simulink model "Quadrotor_model_2020_PID_R2025a"  (R2025a)
settings: Solver=FixedStepDiscrete  StartTime=0.0  StopTime=q2020_t_stop  FixedStep=pid_dt  RelTol=1e-3  EnableMultiTasking=on
InitFcn:
  | run('C:\00_Research_\Neuromorphic_Embodied_AI\02_Coaxial_TriRotor_Nengo\baseline_victor\PID_R2025a_models\params\victor_pid_params.m')
undefined symbols (not defined in the file): pid_dt, q2020_int0, q2020_param_vec, q2020_x0
settings Model: ExtModeTrigDuration=10000  Creator=gandhico  LastModifiedBy=gandhico
settings SolverCC: AlgebraicLoopSolver=TrustRegion  PositivePriorityOrder=on
settings DataIOCC: ReturnWorkspaceOutputs=off
settings DebuggingCC: UnconnectedInputMsg=warning  UnconnectedOutputMsg=warning  UnconnectedLineMsg=warning  ArithmeticOperatorsInVariantConditions=warning
settings ModelReferenceCC: EnableRefExpFcnMdlSchedulingChecks=on
settings SFSimCC: SimUseLocalCustomCode=off  CustomCodeUndefinedFunction=UseInterfaceOnly
settings RTWCC: SystemTargetFile=quarc_win64.tlc  TemplateMakefile=quarc_default_tmf  RTWUseLocalCustomCode=off  Toolchain=QUARC win64 | nmake (64-bit Windows)  BuildConfiguration=Faster Runs  GPUComputeCapability=3.5  Description=QUARC Win64 Target Using Toolchain
settings CodeAppCC: StateflowObjectComments=on
settings STFCustomTargetCC: SystemTargetFile=quarc_win64.tlc  TargetLangStandard=C99 (ISO)  MultiwordLength=2048.0  DynamicStringBufferSize=256.0  ConcurrentExecutionCompliant=on  UseToolchainInfoCompliant=on
settings GRTTargetCC: ExtMode=on  ExtModeMexFile=quarc_comm  ParMdlRefBuildCompliant=off  CompOptLevelCompliant=off  CombineOutputUpdateFcns=off  MatFileLogging=off  CPPClassGenCompliant=off  GRTInterface=on
settings ConfigComp: CovMetricSettings=dswe

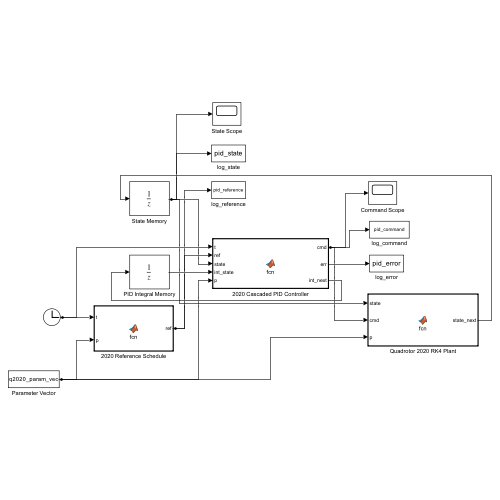
[thumbnail: Simulink's stored preview of the top-level diagram]
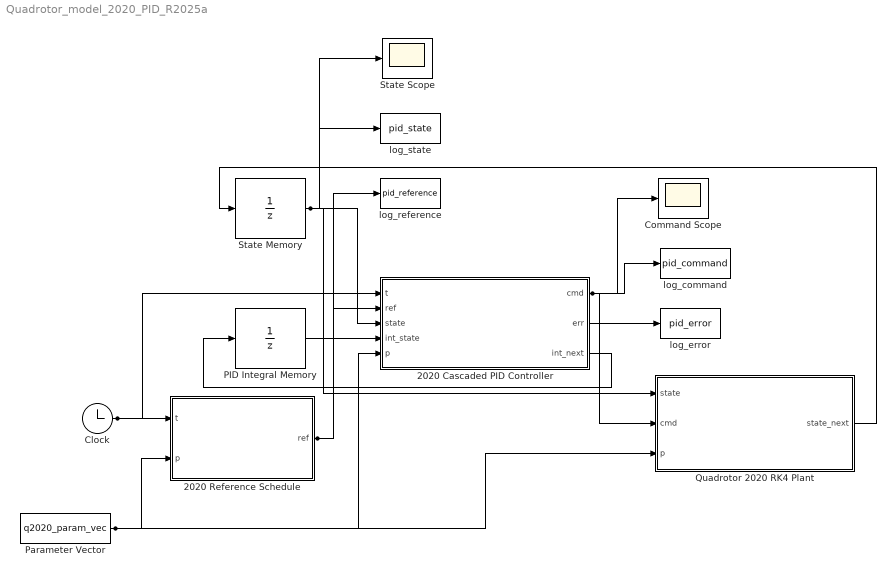
== system Quadrotor_model_2020_PID_R2025a ==
  2020 Cascaded PID Controller : MATLAB Function  TreatAsAtomicUnit=on
  2020 Reference Schedule : MATLAB Function  TreatAsAtomicUnit=on
  Clock : Clock
  Command Scope : Scope
  PID Integral Memory : UnitDelay  InitialCondition=q2020_int0  SampleTime=pid_dt  HasFrameUpgradeWarning=on
  Parameter Vector : Constant  Value=q2020_param_vec
  Quadrotor 2020 RK4 Plant : MATLAB Function  TreatAsAtomicUnit=on
  State Memory : UnitDelay  InitialCondition=q2020_x0  SampleTime=pid_dt  HasFrameUpgradeWarning=on
  State Scope : Scope
  log_command : ToWorkspace  VariableName=pid_command  SaveFormat=Structure With Time  SampleTime=-1
  log_error : ToWorkspace  VariableName=pid_error  SaveFormat=Structure With Time  SampleTime=-1
  log_reference : ToWorkspace  VariableName=pid_reference  SaveFormat=Structure With Time  SampleTime=-1
  log_state : ToWorkspace  VariableName=pid_state  SaveFormat=Structure With Time  SampleTime=-1
  wires:
  2020 Cascaded PID Controller/3(int_next) -> PID Integral Memory/1
  PID Integral Memory/1 -> 2020 Cascaded PID Controller/4(int_state)
  Parameter Vector/1 -> 2020 Cascaded PID Controller/5(p), Quadrotor 2020 RK4 Plant/3(p), 2020 Reference Schedule/2(p)
  Clock/1 -> 2020 Cascaded PID Controller/1(t), 2020 Reference Schedule/1(t)
  State Memory/1 -> log_state/1, Quadrotor 2020 RK4 Plant/1(state), State Scope/1, 2020 Cascaded PID Controller/3(state)
  2020 Reference Schedule/1(ref) -> 2020 Cascaded PID Controller/2(ref), log_reference/1
  2020 Cascaded PID Controller/1(cmd) -> Quadrotor 2020 RK4 Plant/2(cmd), log_command/1, Command Scope/1
  2020 Cascaded PID Controller/2(err) -> log_error/1
  Quadrotor 2020 RK4 Plant/1(state_next) -> State Memory/1

== matlab function Quadrotor_model_2020_PID_R2025a/2020 Cascaded PID Controller ==
  data: t input size=[1 1]; cmd output size=[9 1]; ref input size=[7 1]; state input size=[12 1]; int_state input size=[6 1]; p input size=[32 1]; err output size=[12 1]; int_next output size=[6 1]
function [cmd, err, int_next] = fcn(t, ref, state, int_state, p)
%#codegen
pid_dt = p(1);
m = p(2);
g = p(3);
kp_z = p(5); ki_z = p(6); kd_z = p(7);
kp_x = p(8); ki_x = p(9); kd_x = p(10);
kp_y = p(11); ki_y = p(12); kd_y = p(13);
kp_phi = p(14); ki_phi = p(15); kd_phi = p(16);
kp_psi = p(17); ki_psi = p(18); kd_psi = p(19);
kp_theta = p(20); ki_theta = p(21); kd_theta = p(22);
tilt_limit = p(23);
den_min = p(24);
u_min = p(25);
u_max = p(26);
tau_psi_limit = p(27);
tau_theta_limit = p(28);
tau_phi_limit = p(29);
int_xy_lim = p(30);
int_z_lim = p(31);
int_att_lim = p(32);

x = state(1); dx = state(2);
y = state(3); dy = state(4);
z = state(5); dz = state(6);
psi = state(7); dpsi = state(8);
theta = state(9); dtheta = state(10);
phi = state(11); dphi = state(12);

ex = ref(1) - x;
edx = ref(2) - dx;
ey = ref(3) - y;
edy = ref(4) - dy;
ez = ref(5) - z;
edz = -dz;
epsi = wrap_pi(ref(7) - psi);
edpsi = -dpsi;

integ_new = int_state;
integ_new(1) = sat(int_state(1) + pid_dt*ex, int_xy_lim);
integ_new(2) = sat(int_state(2) + pid_dt*ey, int_xy_lim);
integ_new(3) = sat(int_state(3) + pid_dt*ez, int_z_lim);
integ_new(4) = sat(int_state(4) + pid_dt*epsi, int_att_lim);

ax_cmd = kp_x*ex + ki_x*integ_new(1) + kd_x*edx;
ay_cmd = kp_y*ey + ki_y*integ_new(2) + kd_y*edy;
uz_cmd = kp_z*ez + ki_z*integ_new(3) + kd_z*edz;

theta_d = atan2(ax_cmd, g);
phi_d = atan2(-ay_cmd*cos(theta), g);
theta_d = sat(theta_d, tilt_limit);
phi_d = sat(phi_d, tilt_limit);

etheta = theta_d - theta;
edtheta = -dtheta;
ephi = phi_d - phi;
edphi = -dphi;
integ_new(5) = sat(int_state(5) + pid_dt*etheta, int_att_lim);
integ_new(6) = sat(int_state(6) + pid_dt*ephi, int_att_lim);

u_unsat = (m*g + uz_cmd)/max(cos(theta)*cos(phi), den_min);
u = min(max(u_unsat, u_min), u_max);

tau_psi_unsat = kp_psi*epsi + ki_psi*integ_new(4) + kd_psi*edpsi;
tau_theta_unsat = kp_theta*etheta + ki_theta*integ_new(5) + kd_theta*edtheta;
tau_phi_unsat = kp_phi*ephi + ki_phi*integ_new(6) + kd_phi*edphi;

tau_psi = sat(tau_psi_unsat, tau_psi_limit);
tau_theta = sat(tau_theta_unsat, tau_theta_limit);
tau_phi = sat(tau_phi_unsat, tau_phi_limit);

cmd = [u; tau_psi; tau_theta; tau_phi; theta_d; phi_d; ax_cmd; ay_cmd; uz_cmd];
err = [ex; ey; ez; epsi; etheta; ephi; integ_new(1); integ_new(2); integ_new(3); integ_new(4); integ_new(5); integ_new(6)];
int_next = integ_new;
end

function y = sat(x, lim)
y = min(max(x, -lim), lim);
end

function y = wrap_pi(x)
y = mod(x + pi, 2*pi) - pi;
end

== matlab function Quadrotor_model_2020_PID_R2025a/2020 Reference Schedule ==
  data: t input size=[1 1]; ref output size=[7 1]; p input size=[32 1]
function ref = fcn(t, p)
%#codegen
omega = p(4);
x_ref = sin(omega*t);
dx_ref = omega*cos(omega*t);
y_ref = sin(omega*t);
dy_ref = omega*cos(omega*t);
[z_ref, dz_ref] = z_schedule(t);
psi_ref = 0.0;
ref = [x_ref; dx_ref; y_ref; dy_ref; z_ref; dz_ref; psi_ref];
end

function [z_ref, dz_ref] = z_schedule(t)
if t < 10.0
    z_ref = t/10.0;
    dz_ref = 0.1;
elseif t < 20.0
    z_ref = 1.0;
    dz_ref = 0.0;
elseif t < 30.0
    z_ref = 1.0 + (0.5 - 1.0)*(t - 20.0)/(30.0 - 20.0);
    dz_ref = -0.05;
else
    z_ref = 0.5;
    dz_ref = 0.0;
end
end

== matlab function Quadrotor_model_2020_PID_R2025a/Quadrotor 2020 RK4 Plant ==
  data: state input size=[12 1]; state_next output size=[12 1]; cmd input size=[9 1]; p input size=[32 1]
function state_next = fcn(state, cmd, p)
%#codegen
h = p(1);
k1 = dyn_quad2020(state, cmd, p);
k2 = dyn_quad2020(state + 0.5*h*k1, cmd, p);
k3 = dyn_quad2020(state + 0.5*h*k2, cmd, p);
k4 = dyn_quad2020(state + h*k3, cmd, p);
state_next = state + (h/6.0)*(k1 + 2.0*k2 + 2.0*k3 + k4);
end

function dX = dyn_quad2020(x, cmd, p)
m = p(2);
g = p(3);
u = cmd(1);
tau_psi = cmd(2);
tau_theta = cmd(3);
tau_phi = cmd(4);
psi = x(7); theta = x(9); phi = x(11);

dX = zeros(12,1);
dX(1) = x(2);
dX(2) = u*(sin(phi)*sin(psi) + cos(phi)*cos(psi)*sin(theta))/m;
dX(3) = x(4);
dX(4) = u*(cos(phi)*sin(theta)*sin(psi) - cos(psi)*sin(phi))/m;
dX(5) = x(6);
dX(6) = u*(cos(theta)*cos(phi))/m - g;
dX(7) = x(8);
dX(8) = tau_psi;
dX(9) = x(10);
dX(10) = tau_theta;
dX(11) = x(12);
dX(12) = tau_phi;
end
